simulink model "passivity_control__estimator"  (R2023b)
settings: Solver=VariableStepAuto  StartTime=0.0  StopTime=30.0  RelTol=1e-3
InitFcn:
  | %% INITFNC - Spiral Trajectory
  | %% UAV PARAMETERS
  | mass = 4.34;
  | Ib = diag([0.08, 0.08, 0.14]);
  | run('filtro.m')
  | %% SAMPLING TIME
  | Ts = 0.001;
  | 
  | %% TRAJECTORY SETTINGS
  | t_iniz = 0;
  | ttot = 20;
  | tdead = 10;
  | tot_time = ttot + tdead;
  | t = linspace(0, tot_time, round(tot_time/Ts));
  | 
  | %% TRAJECTORY PARAMETERS
  | omega = 0.4;
  | radius = 1;
  | z_start = 1;
  | z_end = 3;
  | psi_const = deg2rad(0);
  | 
  | 
  | x_d = radius * cos(omega * t);
  | y_d = radius * sin(omega * t);
  | z_d = linspace(z_start, z_end, length(t));
  | psi_d = psi_const * ones(size(t));
  | 
  | 
  | dx_d = -radius * omega * sin(omega * t);
  | dy_d =  radius * omega * cos(omega * t);
  | dz_d = (z_end - z_start)/tot_time * ones(size(t));
  | dot_psi_d = zeros(size(t));
  | 
  | 
  | ddx_d = -radius * omega^2 * cos(omega * t);
  | ddy_d = -radius * omega^2 * sin(omega * t);
  | ddz_d = zeros(size(t));
  | ddot_psi_d = zeros(size(t));
  | 
  | 
  | p_d = [x_d; y_d; z_d; psi_d];
  | dot_p_d = [dx_d; dy_d; dz_d; dot_psi_d];
  | ddot_p_d = [ddx_d; ddy_d; ddz_d; ddot_psi_d];
  | 
  | p_final = p_d(:, end);
  | dot_p_final = dot_p_d(:, end);
  | ddot_p_final = ddot_p_d(:, end);
  | n_dead = round(tdead / Ts);
  | p_d = [p_d, repmat(p_final, 1, n_dead)];
  | dot_p_d = [dot_p_d, repmat(dot_p_final, 1, n_dead)];
  | ddot_p_d = [ddot_p_d, repmat(ddot_p_final, 1, n_dead)];
  | 
  | 
  | target_len = length(t);
  | p_d = p_d(:, 1:target_len);
  | dot_p_d = dot_p_d(:, 1:target_len);
  | ddot_p_d = ddot_p_d(:, 1:target_len);
  | 
  | %% OUTPUTS FOR SIMULINK
  | x0 = p_d(1,1); y0 = p_d(2,1); z0 = p_d(3,1);
  | pos_0 = [x0 y0 z0];
  | lin_vel_0 = [dot_p_d(1,1), dot_p_d(2,1), dot_p_d(3,1)];
  | w_bb_0 = [0 0 0];
  | 
  | csi_d = p_d(1:3,:);
  | dot_csi_d = dot_p_d(1:3,:);
  | ddot_csi_d = ddot_p_d(1:3,:);
  | psi_d = p_d(4,:);
  | dot_psi_d = dot_p_d(4,:);
  | ddot_psi_d = ddot_p_d(4,:);
  | 
  | %%  Butterworth filter
  |  r=3;
  |  [b, a] = butter(r, 5, 'low', 's');  % Butterworth filter of order r
  |  K = zeros(r,1);
  |  prod = 1;
  |  for j = 1:r
  |      K(j) = a(j+1)/prod;
  |     prod = prod*K(j);
  |  end
  |  K = flip(K);
  | 
  |  intv=[];
  |  for i=1:r
  |     v(i).vec = zeros(6,1);
  |      intv = [intv,v(i).vec];
  |  end
libraries: robotcorelib x1, uavutilslib x1
settings Model: Creator=lidia  LastModifiedBy=lidia

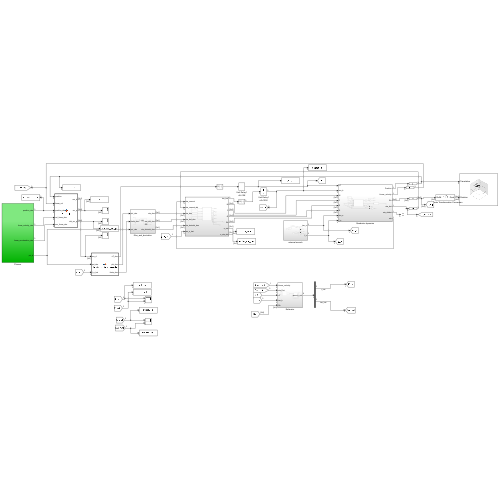
[thumbnail: Simulink's stored preview of the top-level diagram]
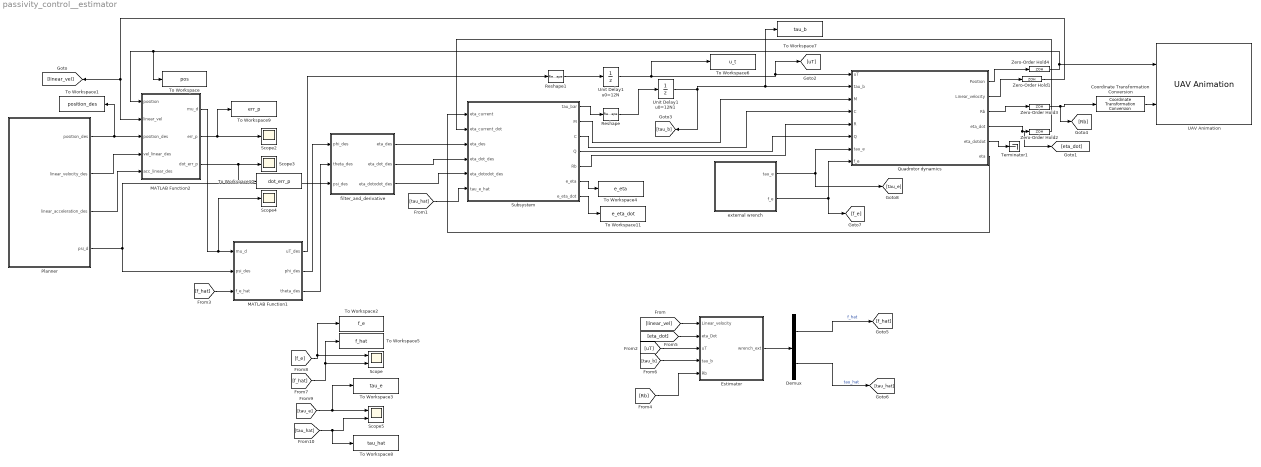
== system passivity_control__estimator ==
  Coordinate Transformation Conversion : robotcorelib/Coordinate Transformation Conversion  InputRepresentation=Rotation Matrix  InputEulerSequence=ZYX  ShowTrVecInputPort=on  OutputRepresentation=Quaternion  OutputEulerSequence=ZYX  ShowTrVecOutputPort=on  SimulateUsing=Interpreted execution
  Demux : Demux  Outputs=2
  Estimator : Subsystem
  MATLAB Function1 : MATLAB Function  TreatAsAtomicUnit=on
  MATLAB Function2 : MATLAB Function  TreatAsAtomicUnit=on
  Planner : Subsystem
  Quadrotor dynamics : Subsystem
  Reshape : Reshape
  Reshape1 : Reshape
  Scope : Scope  NumInputPorts=2
  Scope2 : Scope
  Scope3 : Scope
  Scope4 : Scope
  Scope5 : Scope  NumInputPorts=2
  Subsystem : Subsystem
  Terminator1 : Terminator
  To Workspace : ToWorkspace  VariableName=pos  SaveFormat=Timeseries  SampleTime=-1
  To Workspace1 : ToWorkspace  VariableName=position_des  SaveFormat=Timeseries  SampleTime=-1
  To Workspace10 : ToWorkspace  VariableName=dot_err_p  SaveFormat=Timeseries  SampleTime=-1
  To Workspace11 : ToWorkspace  VariableName=e_eta_dot  SaveFormat=Timeseries  SampleTime=Ts
  To Workspace2 : ToWorkspace  VariableName=f_e  SaveFormat=Timeseries  SampleTime=-1
  To Workspace3 : ToWorkspace  VariableName=tau_e  SaveFormat=Timeseries  SampleTime=-1
  To Workspace4 : ToWorkspace  VariableName=e_eta  SaveFormat=Timeseries  SampleTime=Ts
  To Workspace5 : ToWorkspace  VariableName=f_hat  SaveFormat=Timeseries  SampleTime=-1
  To Workspace6 : ToWorkspace  VariableName=u_t  SaveFormat=Timeseries  SampleTime=Ts
  To Workspace7 : ToWorkspace  VariableName=tau_b  SaveFormat=Timeseries  SampleTime=Ts
  To Workspace8 : ToWorkspace  VariableName=tau_hat  SaveFormat=Timeseries  SampleTime=-1
  To Workspace9 : ToWorkspace  VariableName=err_p  SaveFormat=Timeseries  SampleTime=-1
  UAV Animation : uavutilslib/UAV Animation  UAVType=Multirotor  UAVSize=1  InertialZDirection=Down  SampleTime=0.01
  Unit Delay1 u0=12N : UnitDelay  InitialCondition=12  SampleTime=Ts
  Unit Delay1 u0=12N1 : UnitDelay  InitialCondition=12  SampleTime=Ts
  Zero-Order Hold{1..4} (4 alike) : ZeroOrderHold  SampleTime=Ts
  external wrench : Subsystem
  filter_and_derivative : Subsystem
  wires:
  Coordinate Transformation Conversion/1 -> UAV Animation/2
  Planner/4(psi_d) -> filter_and_derivative/3(psi_des), MATLAB Function1/2(psi_des)
  Unit Delay1 u0=12N/1 -> To Workspace6/1, [uT], Quadrotor dynamics/1(uT)
  MATLAB Function2/3(dot_err_p) -> To Workspace10/1, Scope3/1
  Planner/1(position_des) -> To Workspace1/1, MATLAB Function2/3(position_des)
  Planner/3(linear_acceleration_des) -> MATLAB Function2/5(acc_linear_des)
  Planner/2(linear_velocity_des) -> MATLAB Function2/4(vel_linear_des)
  MATLAB Function1/1(uT_des) -> Reshape1/1
  Zero-Order Hold4/1 -> UAV Animation/1, To Workspace/1, MATLAB Function2/1(position)
  Quadrotor dynamics/2(Linear_velocity) -> Zero-Order Hold1/1
  MATLAB Function2/1(mu_d) -> Scope4/1, MATLAB Function1/1(mu_d)
  Zero-Order Hold1/1 -> [linear_vel], MATLAB Function2/2(linear_vel)
  Quadrotor dynamics/3(Rb) -> Zero-Order Hold3/1
  Quadrotor dynamics/1(Position) -> Zero-Order Hold4/1
  Unit Delay1 u0=12N1/1 -> [tau_b], To Workspace7/1, Quadrotor dynamics/2(tau_b)
  Zero-Order Hold3/1 -> [Rb], Coordinate Transformation Conversion/1
  Quadrotor dynamics/4(eta_dot) -> [eta_dot], Zero-Order Hold2/1
  Quadrotor dynamics/5(eta_dotdot) -> Terminator1/1
  Zero-Order Hold2/1 -> Subsystem/2(eta_current_dot)
  MATLAB Function1/2(phi_des) -> filter_and_derivative/1(phi_des)
  MATLAB Function1/3(theta_des) -> filter_and_derivative/2(theta_des)
  filter_and_derivative/1(eta_des) -> Subsystem/3(eta_des)
  filter_and_derivative/2(eta_dot_des) -> Subsystem/4(eta_dot_des)
  filter_and_derivative/3(eta_dotodot_des) -> Subsystem/5(eta_dotodot_des)
  Subsystem/1(tau_bar) -> Reshape/1
  Subsystem/2(M) -> Quadrotor dynamics/3(M)
  Subsystem/3(C) -> Quadrotor dynamics/4(C)
  Subsystem/4(Q) -> Quadrotor dynamics/6(Q)
  [linear_vel] -> Estimator/1(Linear_velocity)
  [eta_dot] -> Estimator/2(eta_Dot)
  [uT] -> Estimator/3(uT)
  [tau_b] -> Estimator/4(tau_b)
  [Rb] -> Estimator/5(Rb)
  Estimator/1(wrench_ext) -> Demux/1
  Demux/1 -> [f_hat]  "f_hat"
  Demux/2 -> [tau_hat]  "tau_hat"
  [tau_hat] -> Subsystem/6(tau_e_hat)
  Reshape/1 -> Unit Delay1 u0=12N1/1
  Reshape1/1 -> Unit Delay1 u0=12N/1
  Subsystem/5(Rb) -> Quadrotor dynamics/5(R)
  Quadrotor dynamics/6(eta) -> Subsystem/1(eta_current)
  [f_hat] -> MATLAB Function1/3(f_e_hat)
  external wrench/1(tau_e) -> [tau_e], Quadrotor dynamics/7(tau_e)
  external wrench/2(f_e) -> [f_e], Quadrotor dynamics/8(f_e)
  [f_e] -> To Workspace2/1, Scope/1
  [f_hat] -> To Workspace5/1, Scope/2
  [tau_e] -> To Workspace3/1, Scope5/1
  [tau_hat] -> To Workspace8/1, Scope5/2
  Subsystem/6(e_eta) -> To Workspace4/1
  MATLAB Function2/2(err_p) -> To Workspace9/1, Scope2/1
  Subsystem/7(e_eta_dot) -> To Workspace11/1

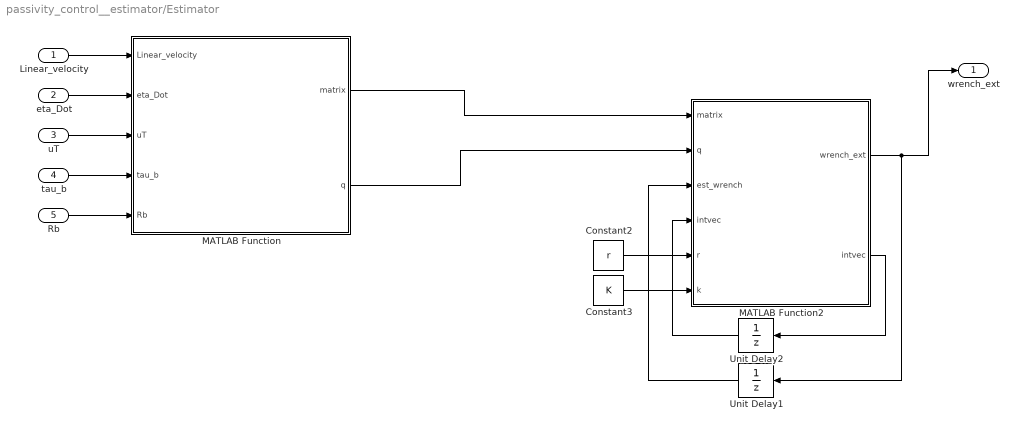
== system passivity_control__estimator/Estimator ==
  Linear_velocity : Inport
  eta_Dot : Inport  Port=2
  uT : Inport  Port=3
  tau_b : Inport  Port=4
  Rb : Inport  Port=5
  Constant2 : Constant  Value=r
  Constant3 : Constant  Value=K
  MATLAB Function : MATLAB Function  TreatAsAtomicUnit=on
  MATLAB Function2 : MATLAB Function  TreatAsAtomicUnit=on
  Unit Delay1 : UnitDelay  InitialCondition=zeros(6,1)  SampleTime=Ts  HasFrameUpgradeWarning=on
  Unit Delay2 : UnitDelay  InitialCondition=intv  SampleTime=Ts  HasFrameUpgradeWarning=on
  wrench_ext : Outport
  wires:
  Linear_velocity/1 -> MATLAB Function/1(Linear_velocity)
  eta_Dot/1 -> MATLAB Function/2(eta_Dot)
  uT/1 -> MATLAB Function/3(uT)
  tau_b/1 -> MATLAB Function/4(tau_b)
  Rb/1 -> MATLAB Function/5(Rb)
  Constant3/1 -> MATLAB Function2/6(k)
  MATLAB Function/2(q) -> MATLAB Function2/2(q)
  MATLAB Function/1(matrix) -> MATLAB Function2/1(matrix)
  MATLAB Function2/2(intvec) -> Unit Delay2/1
  Unit Delay1/1 -> MATLAB Function2/3(est_wrench)
  Constant2/1 -> MATLAB Function2/5(r)
  MATLAB Function2/1(wrench_ext) -> Unit Delay1/1, wrench_ext/1
  Unit Delay2/1 -> MATLAB Function2/4("intvec ")

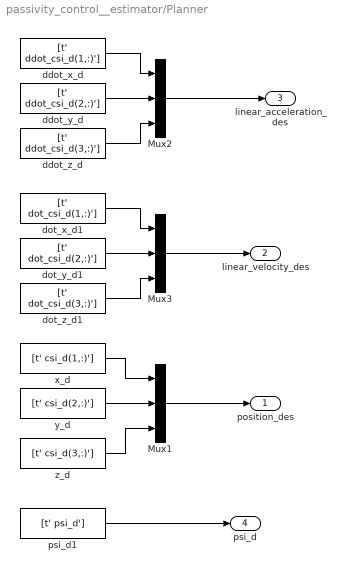
== system passivity_control__estimator/Planner ==
  Mux1 : Mux  Inputs=3
  Mux2 : Mux  Inputs=3
  Mux3 : Mux  Inputs=3
  ddot_x_d : FromWorkspace  VariableName=[t' ddot_csi_d(1,:)']  SampleTime=Ts
  ddot_y_d : FromWorkspace  VariableName=[t' ddot_csi_d(2,:)']  SampleTime=Ts
  ddot_z_d : FromWorkspace  VariableName=[t' ddot_csi_d(3,:)']  SampleTime=Ts
  dot_x_d1 : FromWorkspace  VariableName=[t' dot_csi_d(1,:)']  SampleTime=Ts
  dot_y_d1 : FromWorkspace  VariableName=[t' dot_csi_d(2,:)']  SampleTime=Ts
  dot_z_d1 : FromWorkspace  VariableName=[t' dot_csi_d(3,:)']  SampleTime=Ts
  psi_d1 : FromWorkspace  VariableName=[t' psi_d']  SampleTime=Ts
  x_d : FromWorkspace  VariableName=[t' csi_d(1,:)']  SampleTime=Ts
  y_d : FromWorkspace  VariableName=[t' csi_d(2,:)']  SampleTime=Ts
  z_d : FromWorkspace  VariableName=[t' csi_d(3,:)']  SampleTime=Ts
  position_des : Outport
  linear_velocity_des : Outport  Port=2
  linear_acceleration_des : Outport  Port=3
  psi_d : Outport  Port=4
  wires:
  y_d/1 -> Mux1/2
  z_d/1 -> Mux1/3
  x_d/1 -> Mux1/1
  ddot_y_d/1 -> Mux2/2
  ddot_z_d/1 -> Mux2/3
  ddot_x_d/1 -> Mux2/1
  Mux2/1 -> linear_acceleration_des/1
  Mux1/1 -> position_des/1
  dot_y_d1/1 -> Mux3/2
  dot_z_d1/1 -> Mux3/3
  dot_x_d1/1 -> Mux3/1
  Mux3/1 -> linear_velocity_des/1
  psi_d1/1 -> psi_d/1

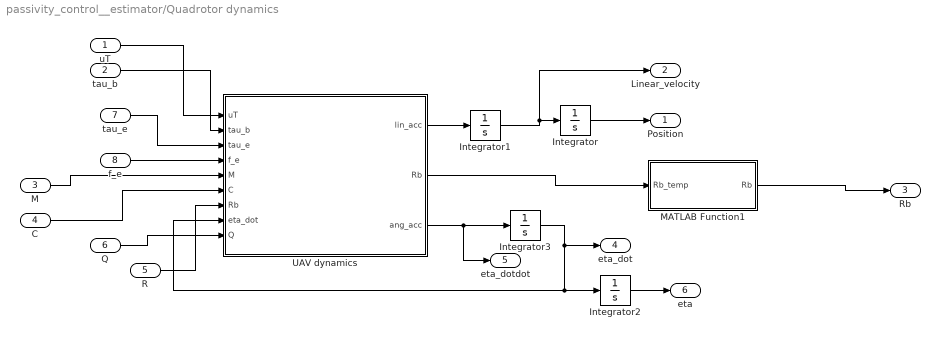
== system passivity_control__estimator/Quadrotor dynamics ==
  uT : Inport
  tau_b : Inport  Port=2
  M : Inport  Port=3
  C : Inport  Port=4
  R : Inport  Port=5
  Q : Inport  Port=6
  tau_e : Inport  Port=7
  f_e : Inport  Port=8
  Integrator : Integrator  InitialCondition=pos_0
  Integrator1 : Integrator  InitialCondition=lin_vel_0
  Integrator2 : Integrator  InitialCondition=w_bb_0
  Integrator3 : Integrator  InitialCondition=w_bb_0
  MATLAB Function1 : MATLAB Function  TreatAsAtomicUnit=on
  UAV dynamics : MATLAB Function  TreatAsAtomicUnit=on
  Position : Outport
  Linear_velocity : Outport  Port=2
  Rb : Outport  Port=3
  eta_dot : Outport  Port=4
  eta_dotdot : Outport  Port=5
  eta : Outport  Port=6
  wires:
  tau_b/1 -> UAV dynamics/2(tau_b)
  Integrator/1 -> Position/1
  UAV dynamics/3(ang_acc) -> eta_dotdot/1, Integrator3/1
  UAV dynamics/1(lin_acc) -> Integrator1/1
  uT/1 -> UAV dynamics/1(uT)
  Integrator1/1 -> Linear_velocity/1, Integrator/1
  MATLAB Function1/1(Rb) -> Rb/1
  M/1 -> UAV dynamics/5(M)
  C/1 -> UAV dynamics/6(C)
  Integrator3/1 -> Integrator2/1, UAV dynamics/8(eta_dot), eta_dot/1
  Q/1 -> UAV dynamics/9(Q)
  R/1 -> UAV dynamics/7("Rb ")
  Integrator2/1 -> eta/1
  UAV dynamics/2(Rb) -> MATLAB Function1/1(Rb_temp)
  tau_e/1 -> UAV dynamics/3(tau_e)
  f_e/1 -> UAV dynamics/4(f_e)

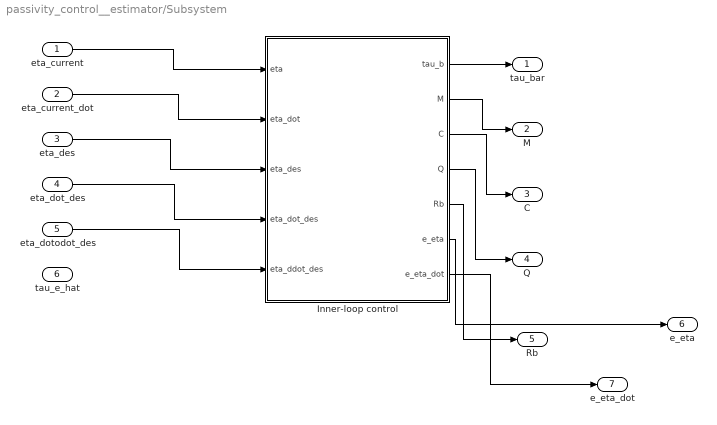
== system passivity_control__estimator/Subsystem ==
  eta_current : Inport
  eta_current_dot : Inport  Port=2
  eta_des : Inport  Port=3
  eta_dot_des : Inport  Port=4
  eta_dotodot_des : Inport  Port=5
  tau_e_hat : Inport  Port=6
  Inner-loop control : MATLAB Function  TreatAsAtomicUnit=on
  tau_bar : Outport
  M : Outport  Port=2
  C : Outport  Port=3
  Q : Outport  Port=4
  Rb : Outport  Port=5
  e_eta : Outport  Port=6
  e_eta_dot : Outport  Port=7
  wires:
  eta_dotodot_des/1 -> Inner-loop control/5(eta_ddot_des)
  eta_current/1 -> Inner-loop control/1(eta)
  eta_current_dot/1 -> Inner-loop control/2(eta_dot)
  eta_des/1 -> Inner-loop control/3(eta_des)
  eta_dot_des/1 -> Inner-loop control/4(eta_dot_des)
  Inner-loop control/1(tau_b) -> tau_bar/1
  Inner-loop control/2(M) -> M/1
  Inner-loop control/3(C) -> C/1
  Inner-loop control/4(Q) -> Q/1
  Inner-loop control/5(Rb) -> Rb/1
  Inner-loop control/6(e_eta) -> e_eta/1
  Inner-loop control/7(e_eta_dot) -> e_eta_dot/1

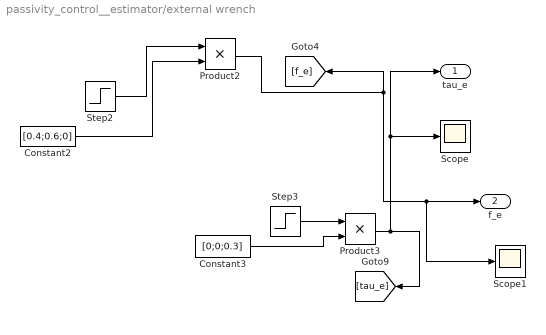
== system passivity_control__estimator/external wrench ==
  Constant2 : Constant  Value=[0.4;0.6;0]  SampleTime=Ts
  Constant3 : Constant  Value=[0;0;0.3]  SampleTime=Ts
  Product2 : Product
  Product3 : Product
  Scope : Scope
  Scope1 : Scope
  Step2 : Step  Time=12  SampleTime=Ts
  Step3 : Step  Time=12  SampleTime=Ts
  tau_e : Outport
  f_e : Outport  Port=2
  wires:
  Constant2/1 -> Product2/2
  Product3/1 -> Scope/1, tau_e/1, [tau_e]
  Product2/1 -> [f_e], Scope1/1, f_e/1
  Step3/1 -> Product3/1
  Step2/1 -> Product2/1
  Constant3/1 -> Product3/2

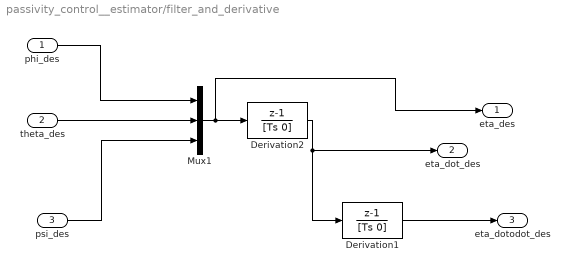
== system passivity_control__estimator/filter_and_derivative ==
  phi_des : Inport
  theta_des : Inport  Port=2
  psi_des : Inport  Port=3
  Derivation1 : DiscreteTransferFcn  Numerator=[1 -1]  Denominator=[Ts 0]  InitialStates=[0 0 0]  SampleTime=Ts
  Derivation2 : DiscreteTransferFcn  Numerator=[1 -1]  Denominator=[Ts 0]  InitialStates=[0 0 0]  SampleTime=Ts
  Mux1 : Mux  Inputs=3
  eta_des : Outport
  eta_dot_des : Outport  Port=2
  eta_dotodot_des : Outport  Port=3
  wires:
  Mux1/1 -> Derivation2/1, eta_des/1
  Derivation1/1 -> eta_dotodot_des/1
  phi_des/1 -> Mux1/1
  theta_des/1 -> Mux1/2
  psi_des/1 -> Mux1/3
  Derivation2/1 -> Derivation1/1, eta_dot_des/1

== matlab function passivity_control__estimator/Estimator/MATLAB Function ==
  data: matrix output; q output; Linear_velocity input; eta_Dot input; uT input; tau_b input; Rb input; mass parameter; Ib parameter
function [matrix, q] = computations(Linear_velocity, eta_Dot, uT, tau_b, Rb, mass, Ib)

q = [mass*eye(3) zeros(3); zeros(3) Ib] * [Linear_velocity; eta_Dot];  %momentum
matrix = [mass*9.81*[0 0 1]'-uT*Rb*[0 0 1]'; -skew(eta_Dot)*Ib*eta_Dot + tau_b];

end
function S = skew(v)
if(numel(v)~= 1)
S= [0 -v(3) v(2); 
    v(3) 0 -v(1);
    -v(2) v(1) 0];
else
S= zeros(3);
end
end

== matlab function passivity_control__estimator/Estimator/MATLAB Function2 ==
  data: matrix input; q input; wrench_ext output; est_wrench input; intvec output; intvec input; r input; k input
function [wrench_ext,intvec] = estimation(matrix,q,est_wrench,intvec,r,k)

    dt=1e-3;
    gamma=zeros(6,r);

    for i=1:r
        if i==1
            intvec(:,i) = intvec(:,i) + (est_wrench+matrix)*dt;
            gamma(:,i) = k(i)*(q-intvec(:,i));
        else
            intvec(:,i) = intvec(:,i) + (-est_wrench+gamma(:,i-1))*dt;
            gamma(:,i) = k(i)*intvec(:,i);
        end
    end
    wrench_ext = gamma(:,r);

end

== matlab function passivity_control__estimator/Quadrotor dynamics/UAV dynamics ==
  data: uT input size=1; tau_b input size=3; tau_e input; f_e input; M input size=[3,3]; C input; lin_acc output size=3; Rb output; Rb input size=[3,3]; eta_dot input; ang_acc output size=3; mass parameter size=1; Q input size=[3,3]
function [lin_acc,Rb, ang_acc] = fcn(uT, tau_b,tau_e,f_e, M, C, Rb, eta_dot, mass, Q)


    lin_acc = 9.81*[0 0 1]' - (uT/mass)*Rb*[0 0 1]' +(1/mass)*f_e;
    
  
    
    ang_acc = inv(M)*(-C*eta_dot + Q'*tau_b + tau_e);

end

function S = skew(v)
if(numel(v)~= 1)
S= [0 -v(3) v(2); 
    v(3) 0 -v(1);
    -v(2) v(1) 0];
else
S= zeros(3);
end
end

== matlab function passivity_control__estimator/MATLAB Function2 ==
  data: position input; mu_d output; linear_vel input; position_des input; vel_linear_des input; acc_linear_des input; err_p output; dot_err_p output
function [mu_d, err_p, dot_err_p] = outerloop(position, linear_vel, ...
    position_des, vel_linear_des, acc_linear_des)

Kp_pos = diag([30, 30, 40]);       
Kd_vel = diag([40, 40, 50]);

err_p     = position - position_des;        
dot_err_p = linear_vel - vel_linear_des;   

proportional_term = Kp_pos * err_p;     

derivative_term   = Kd_vel * dot_err_p;  

mu_d = acc_linear_des - derivative_term - proportional_term;

end

== matlab function passivity_control__estimator/Subsystem/Inner-loop control ==
  data: tau_b output size=3; eta input size=3; eta_dot input size=3; eta_des input size=[3,1]; eta_dot_des input; eta_ddot_des input; Ib parameter; M output; C output; Q output; Rb output; e_eta output; e_eta_dot output
function [tau_b, M,C,Q,Rb,e_eta,e_eta_dot]  = inner_loop_passivity(eta, eta_dot, eta_des, eta_dot_des, eta_ddot_des, Ib)


sigma = 2.3;                   
Ko = diag([30, 30, 30]);       
Do = diag([10, 10, 10]);

e_eta = eta - eta_des;
e_eta_dot = eta_dot - eta_dot_des;

eta_dot_r = eta_dot_des - sigma * e_eta;
eta_ddot_r = eta_ddot_des - sigma * e_eta_dot;


v_eta = e_eta_dot + sigma * e_eta;

% Matrice Q
Q = zeros(3,3);
Q(1,1) = 1;
Q(1,3) = -sin(eta(2));
Q(2,2) = cos(eta(1));
Q(2,3) = cos(eta(2)) * sin(eta(1));
Q(3,2) = -sin(eta(1));
Q(3,3) = cos(eta(2)) * cos(eta(1));
% Derivata di Q
Q_dot = zeros(3,3);
Q_dot(1,3) = -eta_dot(2) * cos(eta(2));
Q_dot(2,2) = -eta_dot(1) * sin(eta(1));
Q_dot(2,3) = -eta_dot(2)*sin(eta(2))*sin(eta(1)) + eta_dot(1)*cos(eta(2))*cos(eta(1));
Q_dot(3,2) = -eta_dot(1)*cos(eta(1));
Q_dot(3,3) = -eta_dot(2)*sin(eta(2))*cos(eta(1)) + eta_dot(1)*cos(eta(2))*sin(eta(1));
% Skew matrix
S = skew(Q * eta_dot);


M = Q' * Ib * Q;
C = Q' * S * Ib * Q + Q' * Ib * Q_dot;
% Rb matrix
Rb = [cos(eta(2))*cos(eta(3)), sin(eta(1))*sin(eta(2))*cos(eta(3)) - cos(eta(1))*sin(eta(3)), cos(eta(1))*sin(eta(2))*cos(eta(3)) + sin(eta(1))*sin(eta(3));
      cos(eta(2))*sin(eta(3)), sin(eta(1))*sin(eta(2))*sin(eta(3)) + cos(eta(1))*cos(eta(3)), cos(eta(1))*sin(eta(2))*sin(eta(3)) - sin(eta(1))*cos(eta(3));
      -sin(eta(2)),            sin(eta(1))*cos(eta(2)),                                      cos(eta(1))*cos(eta(2))];

virtual_command = M * eta_ddot_r + C * eta_dot_r - Do * v_eta - Ko * e_eta;


tau_b = inv(Q') * virtual_command; 

end

function S = skew(v)
if numel(v) == 3
    S = [  0     -v(3)   v(2);
          v(3)    0    -v(1);
         -v(2)  v(1)     0  ];
else
    S = zeros(3,3);
end
end

== matlab function passivity_control__estimator/Quadrotor dynamics/MATLAB Function1 ==
  data: Rb_temp input; Rb output
function Rb = fcn(Rb_temp)
    [U,S,V] = svd(Rb_temp);
    sigma = det(U*V');
    S_ = diag([1 1 sigma]);

    Rb = U*S_*V';
end

== matlab function passivity_control__estimator/MATLAB Function1 ==
  data: mu_d input; uT_des output; psi_des input; phi_des output; theta_des output; mass parameter; f_e_hat input

function [uT_des, phi_des, theta_des] = thrustandattitude_passivity(mu_d, psi_des, mass, f_e_hat)
    
    g = 9.81;
    
    mu_bar = mu_d - (1/mass) * f_e_hat;
  

    mux = mu_bar(1);
    muy = mu_bar(2);
    muz = mu_bar(3);

    
    uT_des = mass * sqrt(mux^2 + muy^2 + (muz - g)^2);
    
    phi_des = asin((-mux * sin(psi_des) + muy * cos(psi_des)) * (mass / uT_des));
    
    theta_des = atan((mux * cos(psi_des) + muy * sin(psi_des)) / (muz - g));
end
